simulink model "m2"  (R2025a)
settings: Solver=VariableStepAuto  StartTime=0.0  StopTime=0.1  RelTol=1e-3
libraries: spsDetailedThyristorLib x4, spsVoltageMeasurementLib x2, spsACVoltageSourceLib x1, spsCurrentMeasurementLib x1, spsSeriesRLCBranchLib x1, spspowerguiLib x1
settings Model: Creator=28097  LastModifiedBy=28097

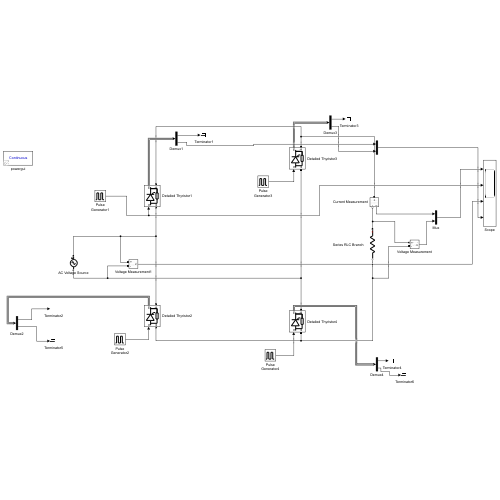
[thumbnail: Simulink's stored preview of the top-level diagram]
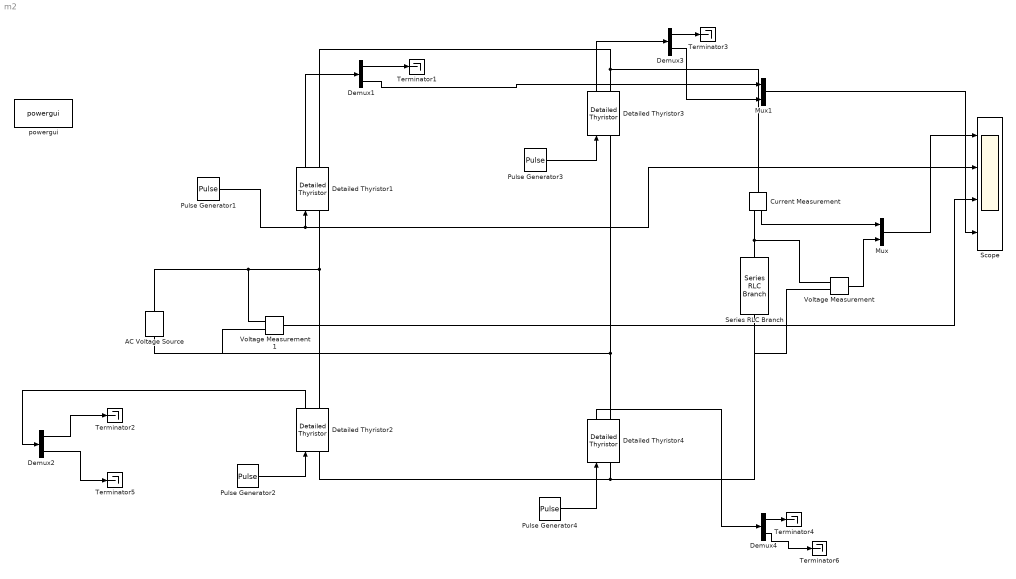
== system m2 ==
  AC Voltage Source : spsACVoltageSourceLib/AC Voltage Source  Amplitude=220*sqrt(3)  Phase=0  Frequency=50  SampleTime=0  Measurements=None  BusType=swing  Pref=10e3  Qref=0  Qmin=-inf  Qmax=+inf
  Current Measurement : spsCurrentMeasurementLib/Current Measurement  PhasorSimulation=off  OutputType=Complex  PSBequivalent=0
  Demux{1..4} (4 alike) : Demux  Outputs=2
  Detailed Thyristor{1..4} (4 alike) : spsDetailedThyristorLib/Detailed Thyristor  Ron=0.001  Lon=1e-3  Vf=0.8  IL=0.1  Tq=100e-6  IC=0  Rs=500  Cs=250e-9  Measurements=on
  Mux : Mux  Inputs=2
  Mux1 : Mux  Inputs=2
  Pulse Generator1 : DiscretePulseGenerator  PulseType=Time based  Amplitude=3  Period=0.02  PulseWidth=10  PhaseDelay=0.02*(30/360)
  Pulse Generator2 : DiscretePulseGenerator  PulseType=Time based  Amplitude=3  Period=0.02  PulseWidth=10  PhaseDelay=0.02*(30/360)+0.01
  Pulse Generator3 : DiscretePulseGenerator  PulseType=Time based  Amplitude=3  Period=0.02  PulseWidth=10  PhaseDelay=0.02*(30/360)+0.01
  Pulse Generator4 : DiscretePulseGenerator  PulseType=Time based  Amplitude=3  Period=0.02  PulseWidth=10  PhaseDelay=0.02*(30/360)
  Scope : Scope  NumInputPorts=4
      settings: ActiveDisplayYMinimum=-47.421920060946327  ActiveDisplayYMaximum=426.79709772464071
  Series RLC Branch : spsSeriesRLCBranchLib/Series RLC Branch  LConnTagsString=__new0  RConnTagsString=__new0  BranchType=R  Resistance=10  Inductance=1e-3  SetiL0=off  InitialCurrent=0  Capacitance=1e-6  Setx0=off  InitialVoltage=0  Measurements=None
  Terminator{1..6} (6 alike) : Terminator
  Voltage Measurement : spsVoltageMeasurementLib/Voltage Measurement  PhasorSimulation=off  OutputType=Complex  PSBequivalent=0
  Voltage Measurement1 : spsVoltageMeasurementLib/Voltage Measurement  PhasorSimulation=off  OutputType=Complex  PSBequivalent=0
  powergui : spspowerguiLib/powergui  Priority=1  SimulationMode=Continuous  SampleTime=50e-6  frequency=60  Iterations=50  frequencyindice=50  Pbase=100e6  ErrMax=1e-4  UnitsV=kV  UnitsW=MW  buscounter=0  FunctionMessages=off  echomessages=off  EnableUseOfTLC=off  CurrentSourceSwitches=off  DisableSnubberDevices=off  DisableRonSwitches=off  DisableVfSwitches=off  DisplayEquations=off  AutomaticDiscreteSolvers=off  SolverType=Tustin/Backward Euler (TBE)  Interpol=off  ExternalGateDelay=off  methode=off  Ts=100  x0status=blocks  SPID=on  SwTol=0  HookPort=off  NonlinearTolerance=1e-4  nMaxIteration=100  ContinueOnMaxIteration=off  RestoreLinks=warning  ResistiveCurrentMeasurement=off  Frange=[0:2:500]  Ylog=off  Xlog=on  ShowGrid=off  save=off  variable=ZData  structure=0  ZoomFFT=off  StartTime=0.0  cycles=1  DisplayStyle=1  fundamental=60  FreqAxis=off  MaxFrequency=1000  frequencyindicesteady=1  RmsSteady=1  display=off
  wires:
  Pulse Generator1/1 -> Scope/2, Detailed Thyristor1/1
  Detailed Thyristor1/1 -> Demux1/1
  Demux1/1 -> Terminator1/1
  Demux2/1 -> Terminator2/1
  Demux2/2 -> Terminator5/1
  Detailed Thyristor2/1 -> Demux2/1
  Pulse Generator2/1 -> Detailed Thyristor2/1
  Pulse Generator3/1 -> Detailed Thyristor3/1
  Detailed Thyristor3/1 -> Demux3/1
  Demux3/1 -> Terminator3/1
  Pulse Generator4/1 -> Detailed Thyristor4/1
  Detailed Thyristor4/1 -> Demux4/1
  Demux4/1 -> Terminator4/1
  Demux4/2 -> Terminator6/1
  Demux1/2 -> Mux1/1
  Demux3/2 -> Mux1/2
  Voltage Measurement/1 -> Mux/2
  Current Measurement/1 -> Mux/1
  Mux/1 -> Scope/1
  Voltage Measurement1/1 -> Scope/3
  Mux1/1 -> Scope/4
  connections:
  AC Voltage Source/RConn1 -- Detailed Thyristor2/RConn1 -- Detailed Thyristor1/LConn1 -- Voltage Measurement1/LConn1
  Detailed Thyristor3/RConn1 -- Current Measurement/LConn1 -- Detailed Thyristor1/RConn1
  Detailed Thyristor2/LConn1 -- Voltage Measurement/LConn2 -- Series RLC Branch/RConn1 -- Detailed Thyristor4/LConn1
  Detailed Thyristor3/LConn1 -- AC Voltage Source/LConn1 -- Voltage Measurement1/LConn2 -- Detailed Thyristor4/RConn1
  Series RLC Branch/LConn1 -- Voltage Measurement/LConn1 -- Current Measurement/RConn1
